simulink model "FOCHCC_of_IM"  (R2023a)
settings: Solver=VariableStepAuto  StartTime=0.0  StopTime=10  RelTol=1e-3
undefined symbols (not defined in the file): DiscIntNeverNeededParam
libraries: slpidlib x2, spsUniversalBridgeLib x1, spsDCVoltageSourceLib x1, spsabctodq0Lib x1, spsdq0toabcLib x1, spsAsynchronousMachineSIUnitsLib x1, spsStairGeneratorLib x1, sps_lib x1
settings Model: Creator=Deepak  LastModifiedBy=Egypt_Laptop
settings SolverCC: AlgebraicLoopSolver=TrustRegion
settings DebuggingCC: UnconnectedInputMsg=warning  UnconnectedOutputMsg=warning  UnconnectedLineMsg=warning
settings ModelReferenceCC: EnableRefExpFcnMdlSchedulingChecks=on
settings SFSimCC: CustomCodeUndefinedFunction=UseInterfaceOnly

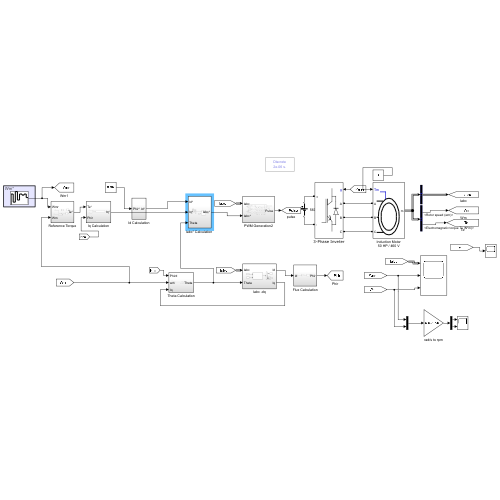
[thumbnail: Simulink's stored preview of the top-level diagram]
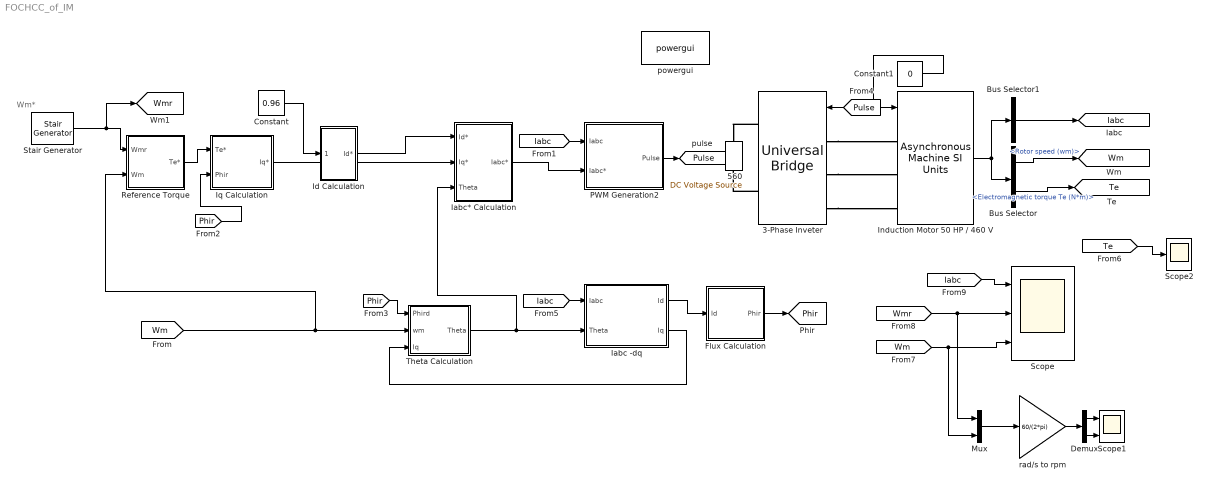
== system FOCHCC_of_IM ==
  note: Wm*
  3-Phase Inveter : spsUniversalBridgeLib/Universal Bridge  Arms=3  SnubberResistance=1e5  SnubberCapacitance=1e-6  Device=IGBT / Diodes  Ron=1e-3  Lon=0  ForwardVoltages="[1.1  0.75]"  ForwardVoltage=0  GTOparameters=[ 10e-6 , 20e-6 ]  IGBTparameters=[ 1e-6 , 2e-6 ]  Measurements=None  Measurements_2=None  converterType=Rectifier
  560 : spsDCVoltageSourceLib/DC Voltage Source  Amplitude=530  Measurements=None
  Bus Selector : BusSelector  OutputSignals=Mechanical.Rotor speed (wm),Mechanical.Electromagnetic torque Te (N*m)
  Bus Selector1 : BusSelector  OutputSignals=Stator measurements.Stator current is_a (A),Stator measurements.Stator current is_b (A),Stator measurements.Stator current is_c (A)  OutputAsBus=on
  Constant : Constant  Value=0.96
  Constant1 : Constant  Value=0
  Demux : Demux  Outputs=2
  Flux Calculation : Subsystem
  Iabc -dq : Subsystem
  "Iabc* Calculation " : Subsystem
  Id Calculation : Subsystem
  Induction Motor 50 HP / 460 V : spsAsynchronousMachineSIUnitsLib/Asynchronous Machine SI Units  RotorType=Squirrel-cage  PresetModel=No  MechanicalLoad=Torque Tm  ShowDetailedParameters=on  ReferenceFrame=Stationary  Units=SI  MeasurementBus=off  NominalParameters=[ 50*746, 460, 60 ]  VoltageRatio=1  Stator=[ 0.087 0.8e-3 ]  Rotor="[ 0.228  0.8e-3 ]"  Cage1=[0.4155 0.002066]  Cage2=[0.4168 0.0003495]  Lm=34.7e-3  Mechanical="[1.662  0.01 2 ]"  PolePairs=2  InitialConditions="[ 1, 0 ,  0 , 0 , 0 , 0 , 0 , 0 ]"  SimulateSaturation=off  Saturation=[0 0;0 0]  LoadFlowParameters=0  TsPowergui=0  TsBlock=-1  IterativeModel=Trapezoidal non iterative  IterativeDiscreteModel=Trapezoidal non iterative  Pmec=1.492e+006
      settings: AttributesFormatString=\n
  Iq Calculation : Subsystem
  Mux : Mux  Inputs=2
  PWM Generation2 : Subsystem
  Reference Torque : Subsystem
  Scope : Scope  NumInputPorts=3
  Scope1 : Scope  NumInputPorts=2
  Scope2 : Scope
  Stair Generator : spsStairGeneratorLib/Stair Generator  t=[0 1 2 3 4 5 6 7 8 9]  e=[50 95 60 105 70 95 90 95 80 55]  Ts=2e-06
  Theta Calculation : Subsystem
  powergui : sps_lib/powergui  Priority=1  SimulationMode=Discrete  SampleTime=2e-6  frequency=60  Iterations=50  frequencyindice=60  Pbase=100e6  ErrMax=1e-4  UnitsV=kV  UnitsW=MW  buscounter=0  FunctionMessages=off  echomessages=off  EnableUseOfTLC=off  CurrentSourceSwitches=off  DisableSnubberDevices=off  DisableRonSwitches=off  DisableVfSwitches=off  DisplayEquations=off  AutomaticDiscreteSolvers=off  SolverType=Tustin/Backward Euler (TBE)  Interpol=off  ExternalGateDelay=off  methode=off  Ts=100  x0status=blocks  SPID=on  SwTol=0  HookPort=off  NonlinearTolerance=0  nMaxIteration=15  ContinueOnMaxIteration=off  RestoreLinks=warning  ResistiveCurrentMeasurement=off  Frange=[0:2:500]  Ylog=off  Xlog=on  ShowGrid=off  save=off  variable=ZData  structure=0  ZoomFFT=off  StartTime=0.0  cycles=1  DisplayStyle=1  fundamental=60  FreqAxis=off  MaxFrequency=1000  frequencyindicesteady=1  RmsSteady=1  display=off
  rad/s to rpm : Gain  Gain=60/(2*pi)
  tag scope: Iabc=global, Phir=global, Pulse=global, Te=global, Wm=global, Wmr=global
  wires:
  Induction Motor 50 HP / 460 V/1 -> Bus Selector/1, Bus Selector1/1
  Bus Selector/1 -> [Wm]  "<Rotor speed (wm)>"
  Bus Selector/2 -> [Te]  "<Electromagnetic torque Te (N*m)>"
  Reference Torque/1(Te*) -> Iq Calculation/1(Te*)
  Iq Calculation/1(Iq*) -> "Iabc* Calculation "/2(Iq*)
  Theta Calculation/1(Theta) -> Iabc -dq/2(Theta), "Iabc* Calculation "/3(Theta)
  Flux Calculation/1(Phir) -> [Phir]
  [Phir] -> Iq Calculation/2(Phir)
  [Iabc] -> Iabc -dq/1(Iabc)
  Id Calculation/1(Id*) -> "Iabc* Calculation "/1(Id*)
  Constant/1 -> Id Calculation/1(Phir*)
  [Wm] -> Mux/2, Scope/3
  [Wmr] -> Scope/2, Mux/1
  [Iabc] -> Scope/1
  Constant1/1 -> Induction Motor 50 HP / 460 V/1
  Bus Selector1/1 -> [Iabc]
  Iabc -dq/1(Id) -> Flux Calculation/1(Id)
  [Phir] -> Theta Calculation/1(Phird)
  [Wm] -> Reference Torque/2(Wm), Theta Calculation/2(wm)
  PWM Generation2/1(Pulse) -> [Pulse]
  Iabc -dq/2(Iq) -> Theta Calculation/3(Iq)
  [Iabc] -> PWM Generation2/1(Iabc)
  [Pulse] -> 3-Phase Inveter/1
  "Iabc* Calculation "/1(Iabc*) -> PWM Generation2/2(Iabc*)
  Stair Generator/1 -> Reference Torque/1(Wmr), [Wmr]
  Demux/1 -> Scope1/1
  Demux/2 -> Scope1/2
  Mux/1 -> rad/s to rpm/1
  rad/s to rpm/1 -> Demux/1
  [Te] -> Scope2/1
  connections:
  3-Phase Inveter/RConn2 -- 560/LConn1
  3-Phase Inveter/LConn1 -- Induction Motor 50 HP / 460 V/LConn1
  3-Phase Inveter/LConn2 -- Induction Motor 50 HP / 460 V/LConn2
  3-Phase Inveter/LConn3 -- Induction Motor 50 HP / 460 V/LConn3
  3-Phase Inveter/RConn1 -- 560/RConn1

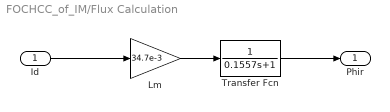
== system FOCHCC_of_IM/Flux Calculation ==
  Id : Inport
  Lm : Gain  Gain=34.7e-3
  Transfer Fcn : TransferFcn  Denominator=[0.1557 1]
  Phir : Outport  VectorParamsAs1DForOutWhenUnconnected=off
  wires:
  Id/1 -> Lm/1
  Lm/1 -> Transfer Fcn/1
  Transfer Fcn/1 -> Phir/1

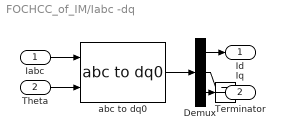
== system FOCHCC_of_IM/Iabc -dq ==
  Iabc : Inport
  Theta : Inport  Port=2
  Demux : Demux  Outputs=3
  Terminator : Terminator
  abc to dq0 : spsabctodq0Lib/abc to dq0  Alignment=90 degrees behind phase A axis
  Id : Outport  VectorParamsAs1DForOutWhenUnconnected=off
  Iq : Outport  Port=2  VectorParamsAs1DForOutWhenUnconnected=off
  wires:
  Demux/3 -> Terminator/1
  abc to dq0/1 -> Demux/1
  Demux/2 -> Iq/1
  Theta/1 -> abc to dq0/2
  Iabc/1 -> abc to dq0/1
  Demux/1 -> Id/1

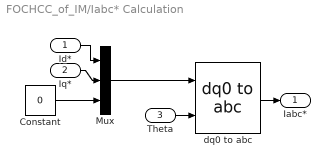
== system FOCHCC_of_IM/Iabc* Calculation  ==
  Id* : Inport
  Iq* : Inport  Port=2
  Theta : Inport  Port=3
  Constant : Constant  Value=0
  Mux : Mux  Inputs=3
  dq0 to abc : spsdq0toabcLib/dq0 to abc  Alignment=90 degrees behind phase A axis
  Iabc* : Outport  VectorParamsAs1DForOutWhenUnconnected=off
  wires:
  dq0 to abc/1 -> Iabc*/1
  Id*/1 -> Mux/1
  Constant/1 -> Mux/3
  Iq*/1 -> Mux/2
  Mux/1 -> dq0 to abc/1
  Theta/1 -> dq0 to abc/2

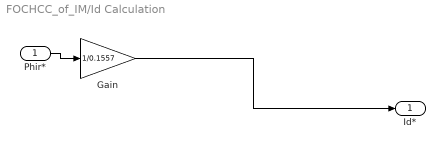
== system FOCHCC_of_IM/Id Calculation ==
  Phir* : Inport
  Gain : Gain  Gain=1/0.1557
  Id* : Outport  VectorParamsAs1DForOutWhenUnconnected=off
  wires:
  Phir*/1 -> Gain/1
  Gain/1 -> Id*/1

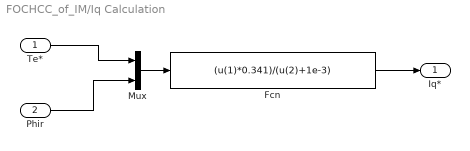
== system FOCHCC_of_IM/Iq Calculation ==
  Te* : Inport
  Phir : Inport  Port=2
  Fcn : Fcn  Expr=(u(1)*0.341)/(u(2)+1e-3)
  Mux : Mux  Inputs=2
  Iq* : Outport  VectorParamsAs1DForOutWhenUnconnected=off
  wires:
  Fcn/1 -> Iq*/1
  Mux/1 -> Fcn/1
  Phir/1 -> Mux/2
  Te*/1 -> Mux/1

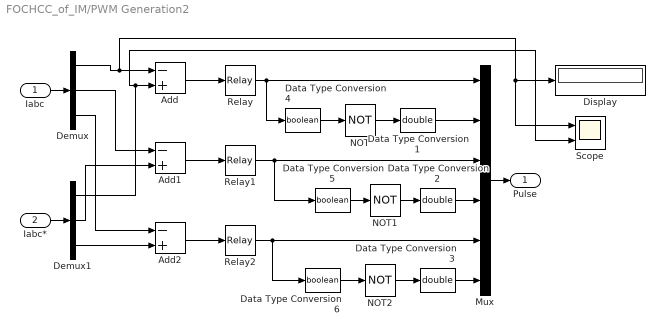
== system FOCHCC_of_IM/PWM Generation2 ==
  Iabc : Inport
  Iabc* : Inport  Port=2
  Add : Sum  Inputs=-+
  Add1 : Sum  Inputs=-+
  Add2 : Sum  Inputs=-+
  Data Type Conversion1 : DataTypeConversion  OutDataTypeStr=double  SaturateOnIntegerOverflow=off  RndMeth=Floor
  Data Type Conversion2 : DataTypeConversion  OutDataTypeStr=double  SaturateOnIntegerOverflow=off  RndMeth=Floor
  Data Type Conversion3 : DataTypeConversion  OutDataTypeStr=double  SaturateOnIntegerOverflow=off  RndMeth=Floor
  Data Type Conversion4 : DataTypeConversion  OutDataTypeStr=boolean  SaturateOnIntegerOverflow=off  RndMeth=Floor
  Data Type Conversion5 : DataTypeConversion  OutDataTypeStr=boolean  SaturateOnIntegerOverflow=off  RndMeth=Floor
  Data Type Conversion6 : DataTypeConversion  OutDataTypeStr=boolean  SaturateOnIntegerOverflow=off  RndMeth=Floor
  Demux : Demux  Outputs=3
  Demux1 : Demux  Outputs=3
  Display : Display
  Mux : Mux  Inputs=6
  NOT : Logic  Operator=NOT  AllPortsSameDT=off  OutDataTypeStr=boolean
  NOT1 : Logic  Operator=NOT  AllPortsSameDT=off  OutDataTypeStr=boolean
  NOT2 : Logic  Operator=NOT  AllPortsSameDT=off  OutDataTypeStr=boolean
  Relay : Relay
  Relay1 : Relay
  Relay2 : Relay
  Scope : Scope  NumInputPorts=2
  Pulse : Outport  VectorParamsAs1DForOutWhenUnconnected=off
  wires:
  Add/1 -> Relay/1
  Relay1/1 -> Data Type Conversion5/1, Mux/3
  NOT/1 -> Data Type Conversion1/1
  Demux1/1 -> Scope/2, Add/2
  Data Type Conversion4/1 -> NOT/1
  Data Type Conversion6/1 -> NOT2/1
  Relay2/1 -> Data Type Conversion6/1, Mux/5
  Mux/1 -> Pulse/1
  Relay/1 -> Data Type Conversion4/1, Mux/1
  Data Type Conversion1/1 -> Mux/2
  Data Type Conversion2/1 -> Mux/4
  Data Type Conversion3/1 -> Mux/6
  Add2/1 -> Relay2/1
  Iabc*/1 -> Demux1/1
  Add1/1 -> Relay1/1
  Data Type Conversion5/1 -> NOT1/1
  NOT2/1 -> Data Type Conversion3/1
  Demux1/2 -> Add1/2
  Demux/2 -> Add1/1
  Demux1/3 -> Add2/2
  Demux/1 -> Scope/1, Display/1, Add/1
  NOT1/1 -> Data Type Conversion2/1
  Demux/3 -> Add2/1
  Iabc/1 -> Demux/1

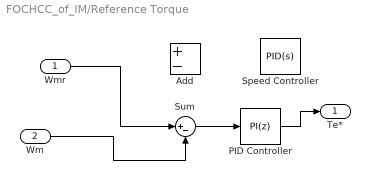
== system FOCHCC_of_IM/Reference Torque ==
  Wmr : Inport
  Wm : Inport  Port=2
  Add : Sum  Inputs=+-
  PID Controller : slpidlib/PID Controller  Controller=PI  Form=Parallel  TimeDomain=Discrete-time  UseExternalTs=off  SampleTime=-1  IntegratorMethod=Forward Euler  FilterMethod=Forward Euler  ControllerParametersSource=internal  P=100  I=26  UseKiTs=off  D=0  N=100  UseFilter=on  TunerSelectOption=Transfer Function Based (PID Tuner App)  InitialConditionSource=internal  InitialConditionForIntegrator=0  InitialConditionForFilter=0  DifferentiatorICPrevScaledInput=0  ExternalReset=none  TrackingMode=off  Kt=1  LimitOutput=off  SatLimitsSource=internal  UpperSaturationLimit=inf  LowerSaturationLimit=-inf  LinearizeAsGain=on  AntiWindupMode=none  Kb=1  LimitIntegrator=off  UpperIntegratorSaturationLimit=inf  LowerIntegratorSaturationLimit=-inf  POutMin=[]  POutMax=[]  IOutMin=[]  IOutMax=[]  DOutMin=[]  DOutMax=[]  NOutMin=[]  NOutMax=[]  SumOutMin=[]  SumOutMax=[]  SaturationOutMin=[]  SaturationOutMax=[]  PParamMin=[]  PParamMax=[]  IParamMin=[]  IParamMax=[]  DParamMin=[]  DParamMax=[]  NParamMin=[]  NParamMax=[]  KbParamMin=[]  KbParamMax=[]  KtParamMin=[]  KtParamMax=[]  KbOutMin=[]  KbOutMax=[]  KtOutMin=[]  KtOutMax=[]  IntegratorOutMin=[]  IntegratorOutMax=[]  FilterOutMin=[]  FilterOutMax=[]  SumI1OutMin=[]  SumI1OutMax=[]  SumI2OutMin=[]  SumI2OutMax=[]  SumI3OutMin=[]  SumI3OutMax=[]  SumI4OutMin=[]  SumI4OutMax=[]  SumDOutMin=[]  SumDOutMax=[]  DifferentiatorOutMin=[]  DifferentiatorOutMax=[]  FilterDiffOutCoefMin=[]  FilterDiffOutCoefMax=[]  ReciprocalOutMin=[]  ReciprocalOutMax=[]  SumDenOutMin=[]  SumDenOutMax=[]  SumNumOutMin=[]  SumNumOutMax=[]  DivideOutMin=[]  DivideOutMax=[]  UdiffTsProdOutMin=[]  UdiffTsProdOutMax=[]  NTsProdOutMin=[]  NTsProdOutMax=[]  UintegralTsProdOutMin=[]  UintegralTsProdOutMax=[]  UngainTsProdOutMin=[]  UngainTsProdOutMax=[]  ClampingZeroOutDataTypeStr=Inherit: Inherit via back propagation  ClampingZeroOutMin=[]  ClampingZeroOutMax=[]  FilterDenConstantOutDataTypeStr=Inherit: Inherit via back propagation  FilterDenConstantOutMin=[]  FilterDenConstantOutMax=[]  PCopyOutDataTypeStr=Inherit: Inherit via back propagation  PCopyOutMin=[]  PCopyOutMax=[]  NCopyOutDataTypeStr=Inherit: Inherit via back propagation  NCopyOutMin=[]  NCopyOutMax=[]  IntegratorContinuousStateAttributes=''  IntegratorStateMustResolveToSignalObject=off  IntegratorRTWStateStorageClass=Auto  FilterContinuousStateAttributes=''  FilterStateMustResolveToSignalObject=off  FilterRTWStateStorageClass=Auto  ParallelPVariant=InternalParameters  IdealPVariant=Disabled  IVariant=InternalParameters  DVariant=Disabled  IntegratorVariant=Discrete  SatVariant=Disabled  AWVariant=Passthrough  PCopyVariant=Disabled  TRVariant=Disabled  FdbkBlocksVariant=Forward  IdealPFdbkVariant=Disabled  SatFdbkVariant=Disabled  DerivativeFilterVariant=Disabled  NVariant=Disabled  NCopyVariant=Disabled_SignalSpec  FilterICVariant=Disabled  IntegratorICVariant=InternalICs  ExternalResetVariant=Disabled  TRSumVariant=Passthrough  SumFdbkVariant=Disabled  SumVariant=Sum_PI  TsampFilterVariant=InternalTs  TsampNgainVariant=Passthrough  TsampIntegralVariant=Disabled_SignalSpec  ExternalSaturationOutDataTypeStr=Inherit: Same as second input
  Speed Controller : slpidlib/PID Controller  Controller=PID  Form=Parallel  TimeDomain=Continuous-time  UseExternalTs=off  SampleTime=2e-6  IntegratorMethod=Forward Euler  FilterMethod=Forward Euler  ControllerParametersSource=internal  P=13  I=26  UseKiTs=off  D=0  N=100  UseFilter=on  TunerSelectOption=Transfer Function Based (PID Tuner App)  InitialConditionSource=internal  InitialConditionForIntegrator=50  InitialConditionForFilter=0  DifferentiatorICPrevScaledInput=0  ExternalReset=none  TrackingMode=off  Kt=1  LimitOutput=on  SatLimitsSource=internal  UpperSaturationLimit=200  LowerSaturationLimit=-200  LinearizeAsGain=off  AntiWindupMode=clamping  Kb=1  LimitIntegrator=off  UpperIntegratorSaturationLimit=inf  LowerIntegratorSaturationLimit=-inf  POutMin=[]  POutMax=[]  IOutMin=[]  IOutMax=[]  DOutMin=[]  DOutMax=[]  NOutMin=[]  NOutMax=[]  SumOutMin=[]  SumOutMax=[]  SaturationOutMin=[]  SaturationOutMax=[]  PParamMin=[]  PParamMax=[]  IParamMin=[]  IParamMax=[]  DParamMin=[]  DParamMax=[]  NParamMin=[]  NParamMax=[]  KbParamMin=[]  KbParamMax=[]  KtParamMin=[]  KtParamMax=[]  KbOutMin=[]  KbOutMax=[]  KtOutMin=[]  KtOutMax=[]  IntegratorOutMin=[]  IntegratorOutMax=[]  FilterOutMin=[]  FilterOutMax=[]  SumI1OutMin=[]  SumI1OutMax=[]  SumI2OutMin=[]  SumI2OutMax=[]  SumI3OutMin=[]  SumI3OutMax=[]  SumI4OutMin=[]  SumI4OutMax=[]  SumDOutMin=[]  SumDOutMax=[]  DifferentiatorOutMin=[]  DifferentiatorOutMax=[]  FilterDiffOutCoefMin=[]  FilterDiffOutCoefMax=[]  ReciprocalOutMin=[]  ReciprocalOutMax=[]  SumDenOutMin=[]  SumDenOutMax=[]  SumNumOutMin=[]  SumNumOutMax=[]  DivideOutMin=[]  DivideOutMax=[]  UdiffTsProdOutMin=[]  UdiffTsProdOutMax=[]  NTsProdOutMin=[]  NTsProdOutMax=[]  UintegralTsProdOutMin=[]  UintegralTsProdOutMax=[]  UngainTsProdOutMin=[]  UngainTsProdOutMax=[]  ClampingZeroOutDataTypeStr=Inherit: Inherit via back propagation  ClampingZeroOutMin=[]  ClampingZeroOutMax=[]  FilterDenConstantOutDataTypeStr=Inherit: Inherit via back propagation  FilterDenConstantOutMin=[]  FilterDenConstantOutMax=[]  PCopyOutDataTypeStr=Inherit: Inherit via back propagation  PCopyOutMin=[]  PCopyOutMax=[]  NCopyOutDataTypeStr=Inherit: Inherit via back propagation  NCopyOutMin=[]  NCopyOutMax=[]  IntegratorContinuousStateAttributes=''  IntegratorStateMustResolveToSignalObject=off  IntegratorRTWStateStorageClass=Auto  FilterContinuousStateAttributes=''  FilterStateMustResolveToSignalObject=off  FilterRTWStateStorageClass=Auto  ParallelPVariant=InternalParameters  IdealPVariant=Disabled  IVariant=InternalParameters  DVariant=InternalParameters  IntegratorVariant=Continuous  SatVariant=Enabled  AWVariant=ContClampingParallel  PCopyVariant=Disabled  TRVariant=Disabled  FdbkBlocksVariant=Forward  IdealPFdbkVariant=Disabled  SatFdbkVariant=Disabled  DerivativeFilterVariant=ContFilter  NVariant=InternalParameters  NCopyVariant=Disabled  FilterICVariant=InternalICsFilter  IntegratorICVariant=InternalICs  ExternalResetVariant=Disabled  TRSumVariant=Passthrough  SumFdbkVariant=Disabled  SumVariant=Sum_PID  TsampFilterVariant=InternalTs  TsampNgainVariant=Passthrough  TsampIntegralVariant=Disabled_SignalSpec  ExternalSaturationOutDataTypeStr=Inherit: Same as second input
  Sum : Sum  Inputs=|+-
  Te* : Outport  VectorParamsAs1DForOutWhenUnconnected=off
  wires:
  Wmr/1 -> Sum/1
  Wm/1 -> Sum/2
  Sum/1 -> PID Controller/1
  PID Controller/1 -> Te*/1

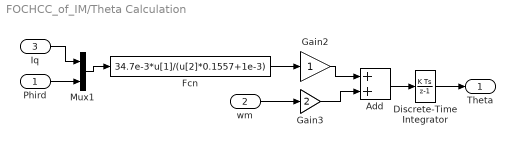
== system FOCHCC_of_IM/Theta Calculation ==
  Phird : Inport
  wm : Inport  Port=2
  Iq : Inport  Port=3
  Add : Sum
  Discrete-Time Integrator : DiscreteIntegrator  SampleTime=1e-5  ICPrevOutput=DiscIntNeverNeededParam  ICPrevScaledInput=DiscIntNeverNeededParam
  Fcn : Fcn  Expr=34.7e-3*u[1]/(u[2]*0.1557+1e-3)
  Gain2 : Gain  SaturateOnIntegerOverflow=on  OutDataTypeStr=Inherit: Same as input  ParamDataTypeStr=Inherit: Same as input
  Gain3 : Gain  Gain=2  SaturateOnIntegerOverflow=on  OutDataTypeStr=Inherit: Same as input  ParamDataTypeStr=Inherit: Same as input
  Mux1 : Mux  Inputs=2
  Theta : Outport  InitialOutput=0  VectorParamsAs1DForOutWhenUnconnected=off
  wires:
  Fcn/1 -> Gain2/1
  Gain3/1 -> Add/2
  wm/1 -> Gain3/1
  Add/1 -> Discrete-Time Integrator/1
  Discrete-Time Integrator/1 -> Theta/1
  Gain2/1 -> Add/1
  Phird/1 -> Mux1/2
  Mux1/1 -> Fcn/1
  Iq/1 -> Mux1/1
